simulink model "MechanicalParameterEstimation"  (R2019b)
settings: Solver=VariableStepAuto  StartTime=0.0  StopTime=1.5*ramp_time  RelTol=1e-3
PreLoadFcn:
  | modelDir = fileparts(get_param(bdroot, 'FileName'));
  | addpath(fullfile(modelDir,'../Parameters'));
  | addpath(fullfile(modelDir,'subsystems'));
  | 
  | Parameters_Model
  | Parameters_Simulation
  | Parameters_Test_Ramp
InitFcn:
  | Parameters_Model
  | Parameters_Simulation
  | Parameters_Test_Ramp
undefined symbols (not defined in the file): n_gear, ramp_duty_end, ramp_duty_start, ramp_steps, ramp_time, Vbat
libraries: simulink x4
settings Model: Creator=Thomas  LastModifiedBy=thomas.jespersen
settings DataIOCC: ReturnWorkspaceOutputs=off
settings DebuggingCC: ArithmeticOperatorsInVariantConditions=warning
settings SFSimCC: SimUseLocalCustomCode=off  CustomCodeUndefinedFunction=UseInterfaceOnly
settings RTWCC: RTWUseLocalCustomCode=off

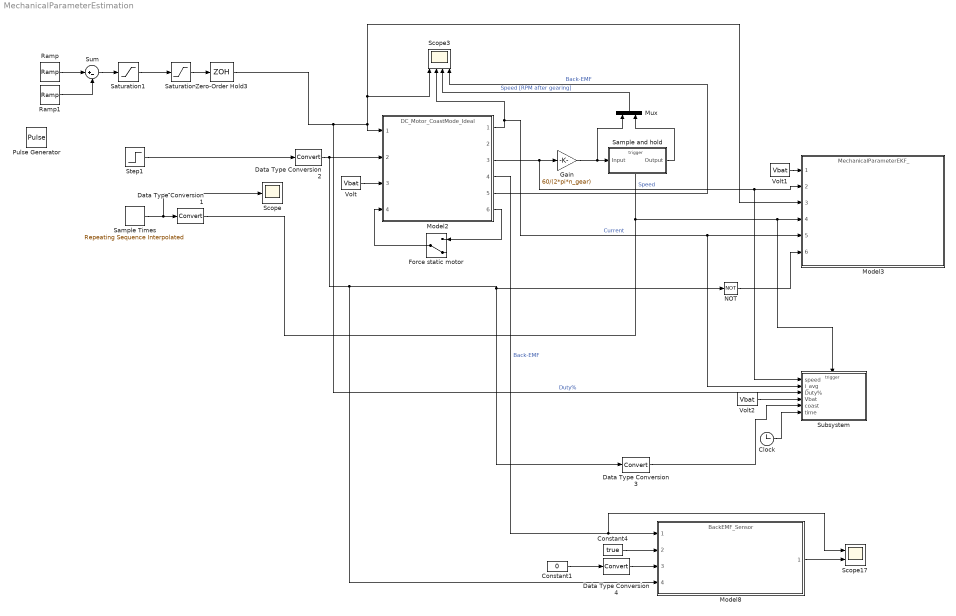
== system MechanicalParameterEstimation ==
  Clock : Clock
  Constant1 : Constant  Value=0
  Constant4 : Constant  Value=true
  Data Type Conversion{1..4} (4 alike) : DataTypeConversion  RndMeth=Round
  Force static motor : ManualSwitch  CurrentSetting=0
  Gain : Gain  Gain=60/(2*pi*n_gear)
  Model2 : ModelReference  ModelNameDialog=DC_Motor_CoastMode_Ideal.slx  SimulationMode=Normal  ModelReferenceVersion=1.31
  Model3 : ModelReference  ModelNameDialog=MechanicalParameterEKF_  SimulationMode=Normal  ModelReferenceVersion=1.63
  Model8 : ModelReference  ModelNameDialog=BackEMF_Sensor  SimulationMode=Normal  ModelReferenceVersion=1.18
  Mux : Mux  Inputs=2
  NOT : Logic  Operator=NOT  IconShape=distinctive  AllPortsSameDT=off  OutDataTypeStr=boolean
  Pulse Generator : DiscretePulseGenerator  PulseType=Time based  Period=8  PulseWidth=50
  Ramp : simulink/Sources/Ramp  slope=(ramp_duty_end-ramp_duty_start)/((ramp_time/ramp_steps)*(ramp_steps-1))  start=0  InitialOutput=ramp_duty_start
  Ramp1 : simulink/Sources/Ramp  slope=2*(ramp_duty_end-ramp_duty_start)/((ramp_time/ramp_steps)*(ramp_steps-1))  start=ramp_time  InitialOutput=0
  Sample Times : simulink/Sources/Repeating Sequence Interpolated  OutValues=ramp_sample_times_signal  TimeValues=ramp_sample_times_t  LookUpMeth=Use Input Below  tsamp=0.001  OutMin=[]  OutMax=[]  OutDataTypeStr=double  OutputDataTypeScalingMode=double  OutDataType=fixdt(0,8)  OutScaling=2^-10
  Sample and hold : Subsystem
  Saturation : Saturate  UpperLimit=1  LowerLimit=-1
  Saturation1 : Saturate  UpperLimit=max(ramp_duty_start, ramp_duty_end)  LowerLimit=min(ramp_duty_start, ramp_duty_end)
  Scope : Scope
  Scope17 : Scope  NumInputPorts=2
  Scope3 : Scope  NumInputPorts=4
  Step1 : Step  Time=ramp_time  Before=1  After=0  SampleTime=0
  Subsystem : Subsystem
  Sum : Sum  Inputs=|+-
  Volt : Constant  Value=Vbat
  Volt1 : Constant  Value=Vbat
  Volt2 : Constant  Value=Vbat
  Zero-Order Hold3 : ZeroOrderHold  SampleTime=ramp_time/(ramp_steps+1)
  wires:
  Volt/1 -> Model2/3
  Force static motor/1 -> Model2/4
  Model2/6 -> Force static motor/1
  Model2/1 -> Subsystem/2(i_avg), Model3/5, Scope3/2  "Current"
  Gain/1 -> Mux/1, Sample and hold/1(Input)
  Step1/1 -> Data Type Conversion2/1
  Data Type Conversion2/1 -> Model8/4, Data Type Conversion3/1, NOT/1, Model2/2
  Model2/5 -> Scope3/4  "Back-EMF"
  Model2/3 -> Subsystem/1(speed), Model3/2, Gain/1  "Speed"
  Sample Times/1 -> Scope/1, Data Type Conversion1/1
  Mux/1 -> Scope3/3  "Speed [RPM after gearing]"
  Sample and hold/1(Output) -> Mux/2
  Volt1/1 -> Model3/1
  Data Type Conversion1/1 -> Model3/4, Subsystem/Trigger, Sample and hold/Trigger
  Ramp/1 -> Sum/1
  Saturation/1 -> Zero-Order Hold3/1
  Volt2/1 -> Subsystem/4(Vbat)
  Data Type Conversion3/1 -> Subsystem/5(coast)
  Clock/1 -> Subsystem/6(time)
  Model8/1 -> Scope17/2
  Constant4/1 -> Model8/2
  Model2/4 -> Scope17/1, Model8/1  "Back-EMF"
  Constant1/1 -> Data Type Conversion4/1
  Data Type Conversion4/1 -> Model8/3
  NOT/1 -> Model3/6
  Zero-Order Hold3/1 -> Subsystem/3(Duty%), Model2/1, Scope3/1, Model3/3  "Duty%"
  Sum/1 -> Saturation1/1
  Ramp1/1 -> Sum/2
  Saturation1/1 -> Saturation/1

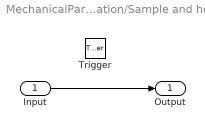
== system MechanicalParameterEstimation/Sample and hold ==
  Input : Inport
  Trigger : TriggerPort  VariantControl=Variant  PortDimensions=1
  Output : Outport  VectorParamsAs1DForOutWhenUnconnected=off
  wires:
  Input/1 -> Output/1

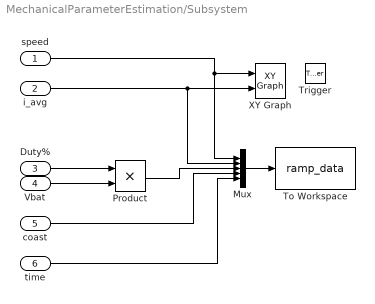
== system MechanicalParameterEstimation/Subsystem ==
  speed : Inport
  i_avg : Inport  Port=2
  Duty% : Inport  Port=3  OutDataTypeStr=double
  Vbat : Inport  Port=4  OutDataTypeStr=double
  coast : Inport  Port=5  OutDataTypeStr=double
  time : Inport  Port=6  OutDataTypeStr=double
  Trigger : TriggerPort  VariantControl=Variant  PortDimensions=1
  Mux : Mux  Inputs=5
  Product : Product
  To Workspace : ToWorkspace  VariableName=ramp_data  SampleTime=-1
      settings: Save2DSignal=2-D array (concatenate along first dimension)
  XY Graph : simulink/Sinks/XY Graph  xmin=0  xmax=1200  ymin=0  ymax=1  st=-1
  wires:
  speed/1 -> XY Graph/1, Mux/1
  i_avg/1 -> Mux/2, XY Graph/2
  Mux/1 -> To Workspace/1
  Vbat/1 -> Product/2
  Duty%/1 -> Product/1
  Product/1 -> Mux/3
  coast/1 -> Mux/4
  time/1 -> Mux/5
